simulink model "SystemModel_Working_wIntegral"  (R2014a)
settings: Solver=ode45  StartTime=0.0  StopTime=30  RelTol=1e-3
values from neighbouring files (symbols this model uses):
  a = 0.92    [SystemModelParameters_Working.m]    (also in SystemModelParameters_wIntegral_Working.m)
  b = 0.5    [SystemModelParameters_Working.m]    (also in SystemModelParameters_wIntegral_Working.m)
  initial = [10,10]    [SystemModelParameters_Working.m]    (also in SystemModelParameters_wIntegral_Working.m)
  J = 6689.281*10^-6    (= 0.006689281)    [PIDTest.m]    (also in SystemModelParameters_Working.m; SystemModelParameters_wIntegral_Working.m)
  kp = 0.0038    [PIDTest.m]    (also in SystemModelParameters_Working.m = 0.4; SystemModelParameters_wIntegral_Working.m = 0.4)
  L = (G/(1+G))    [PIDTest.m]    (also in SystemModelParameters_Working.m = 0.28484; SystemModelParameters_wIntegral_Working.m = 0.28484)
  n = 0    [PIDTest.m]    (also in SystemModelParameters_Working.m = 0.01; SystemModelParameters_wIntegral_Working.m = 0.01)
  PWMs_fixed = [1619,1638]    [SystemModelParameters_Working.m]    (also in SystemModelParameters_wIntegral_Working.m)
  Td = 2.1761/kp    (= 572.657894737)    [PIDTest.m]    (also in SystemModelParameters_Working.m = 0.578; SystemModelParameters_wIntegral_Working.m = 0.578)
  Ti = 1.1    [SystemModelParameters_wIntegral_Working.m]
  Ts = 0.02    [SystemModelParameters_wIntegral_Working.m]
undefined symbols (not defined in the file or in its folder): sigbuilder_block
libraries: aerolibconvert2 x2
settings Model: Creator=lorem  LastModifiedBy=lorem

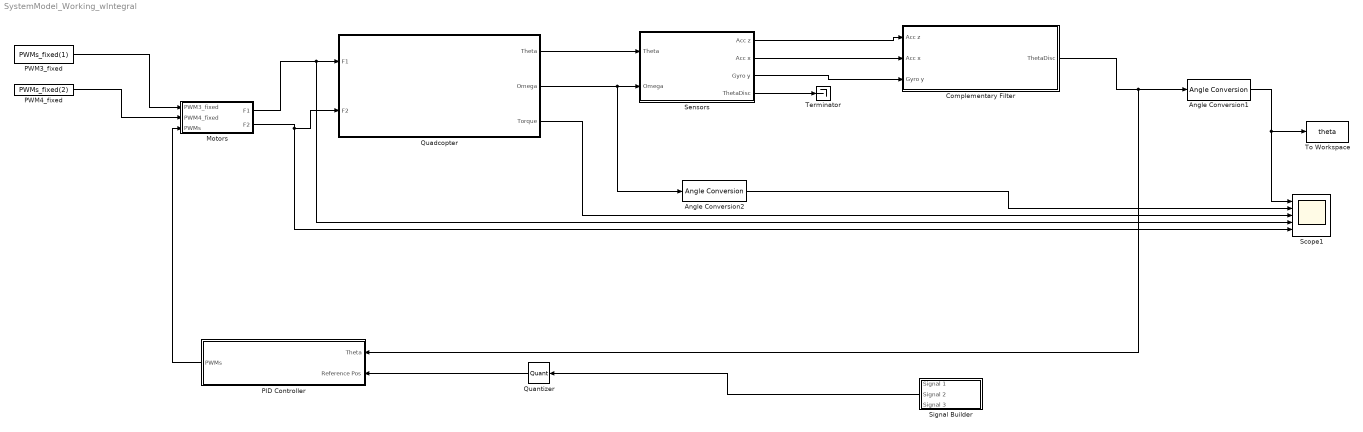
== system SystemModel_Working_wIntegral ==
  Angle Conversion1 : aerolibconvert2/Angle Conversion  IU=rad  OU=deg
  Angle Conversion2 : aerolibconvert2/Angle Conversion  IU=rad  OU=deg
  Complementary Filter : Subsystem
  Motors : Subsystem
  PID Controller : Subsystem
  PWM3_fixed : Constant  Value=PWMs_fixed(1)  SampleTime=0.02
  PWM4_fixed : Constant  Value=PWMs_fixed(2)  SampleTime=0.02
  Quadcopter : Subsystem
  Quantizer : Quantizer  QuantizationInterval=0.01  SampleTime=0.02
  Scope1 : Scope  NumInputPorts=5
      settings: TimeRange=30  YMin=-5~-5~-5~-5~-5  YMax=5~5~5~5~5
  Sensors : Subsystem
  Signal Builder : Subsystem  Tag=STV Subsys  LoadFcn=sigbuilder_block('load');  StartFcn=sigbuilder_block('start');  StopFcn=sigbuilder_block('stop');  ClipboardFcn=sigbuilder_block('clipboard');  mask(Sigbuilder block){}
      mask help: Simulink:masks:SigbuilderBlock_MD
      mask init:
      | if ~strcmp(get_param(bdroot(gcbh),'SimulationStatus'),'stopped') tuvar = sigbuilder_block('maskInit'); end
      settings: CopyFcn=sigbuilder_block('copy');  DeleteFcn=sigbuilder_block('delete');  ModelCloseFcn=sigbuilder_block('modelClose');  PreSaveFcn=sigbuilder_block('preSave');  PauseFcn=sigbuilder_block('pause');  ContinueFcn=sigbuilder_block('continue');  NameChangeFcn=sigbuilder_block('namechange');  OpenFcn=sigbuilder_block('open',[6.75 6.75 1138.5 568.5 ]);  CloseFcn=sigbuilder_block('close');
      mask Display: plot(0, 0, 100, 100,[2, 2, 32, 32, 2], [68, 8, 8, 68, 68],[32, 2], [38, 38], [32, 19, 2],[53, 60, 44], [32, 17, 17, 2],[16, 16, 31, 31]);txt = getActiveGroup(gcbh);text(2, 100, txt,'verticalAlignment', 'top');
  Terminator : Terminator
  To Workspace : ToWorkspace  VariableName=theta  SaveFormat=Timeseries  SampleTime=-1
  wires:
  PWM4_fixed/1 -> Motors/2(PWM4_fixed)
  Motors/2(F2) -> Scope1/5, Quadcopter/2(F2)
  Motors/1(F1) -> Scope1/4, Quadcopter/1(F1)
  Sensors/3(Gyro y) -> Complementary Filter/3(Gyro y)
  Sensors/2(Acc x) -> Complementary Filter/2("Acc x ")
  Sensors/1(Acc z) -> Complementary Filter/1(Acc z)
  PWM3_fixed/1 -> Motors/1(PWM3_fixed)
  PID Controller/1(PWMs) -> Motors/3(PWMs)
  Angle Conversion1/1 -> Scope1/1, To Workspace/1
  Quadcopter/2(Omega) -> Angle Conversion2/1, Sensors/2(Omega)
  Quadcopter/1(Theta) -> Sensors/1(Theta)
  Quadcopter/3("Torque ") -> Scope1/3
  Signal Builder/2(Signal 2) -> Quantizer/1
  Quantizer/1 -> PID Controller/2(Reference Pos)
  Sensors/4(ThetaDisc) -> Terminator/1
  Complementary Filter/1(ThetaDisc) -> PID Controller/1("Theta "), Angle Conversion1/1
  Angle Conversion2/1 -> Scope1/2

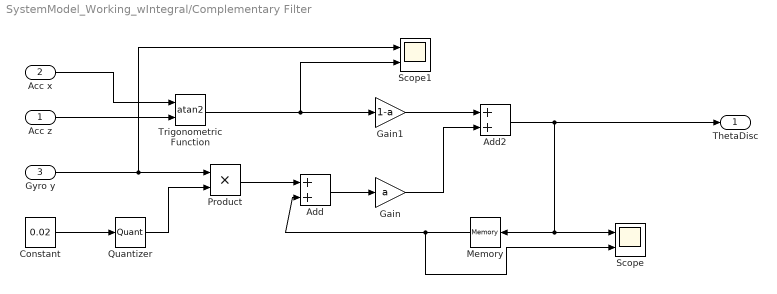
== system SystemModel_Working_wIntegral/Complementary Filter ==
  Acc z : Inport
  "Acc x " : Inport  Port=2
  Gyro y : Inport  Port=3
  Add : Sum
  Add2 : Sum
  Constant : Constant  Value=0.02
  Gain : Gain  Gain=a
  Gain1 : Gain  Gain=1-a
  Memory : Memory  X0=deg2rad(initial(2))  InheritSampleTime=on  LinearizeAsDelay=on
  Product : Product
  Quantizer : Quantizer  QuantizationInterval=0.01  SampleTime=0.02
  Scope : Scope  NumInputPorts=2
      settings: YMin=-5~-5  YMax=5~5  SaveName=ScopeData4
  Scope1 : Scope  NumInputPorts=2
      settings: YMin=-5~-5  YMax=5~5  SaveName=ScopeData5
  Trigonometric Function : Trigonometry  Operator=atan2
  ThetaDisc : Outport
  wires:
  "Acc x "/1 -> Trigonometric Function/1
  Acc z/1 -> Trigonometric Function/2
  Constant/1 -> Quantizer/1
  Gyro y/1 -> Scope1/1, Product/1
  Quantizer/1 -> Product/2
  Product/1 -> Add/1
  Add/1 -> Gain/1
  Gain1/1 -> Add2/1
  Gain/1 -> Add2/2
  Add2/1 -> ThetaDisc/1, Scope/1, Memory/1
  Memory/1 -> Scope/2, Add/2
  Trigonometric Function/1 -> Gain1/1, Scope1/2

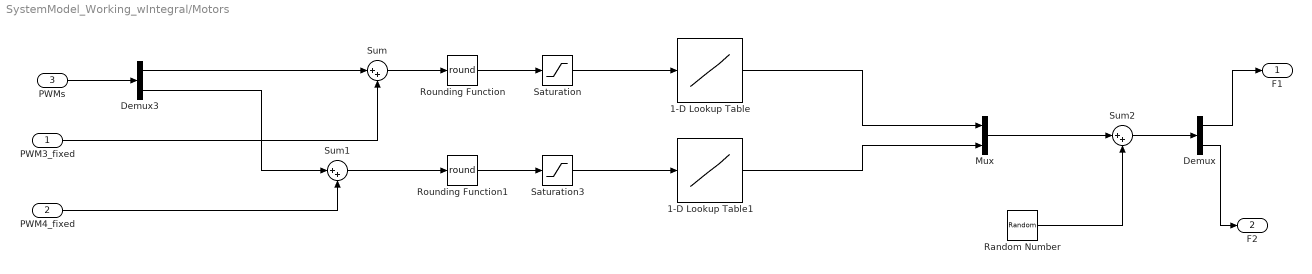
== system SystemModel_Working_wIntegral/Motors ==
  PWM3_fixed : Inport
  PWM4_fixed : Inport  Port=2
  PWMs : Inport  Port=3
  1-D Lookup Table : Lookup_n-D  NumberOfTableDimensions=1  BreakpointsForDimension1=[1447,1792]  Table=[1,5]  InternalRulePriority=Speed  RndMeth=Simplest  InputSameDT=on
  1-D Lookup Table1 : Lookup_n-D  NumberOfTableDimensions=1  BreakpointsForDimension1=[1455,1832]  Table=[1,5]  InternalRulePriority=Speed  RndMeth=Simplest  InputSameDT=on
  Demux : Demux  Outputs=2
  Demux3 : Demux  Outputs=2
  Mux : Mux  Inputs=2
  Random Number : RandomNumber  Variance=0.036579  SampleTime=0.02
  Rounding Function : Rounding  Operator=round
  Rounding Function1 : Rounding  Operator=round
  Saturation : Saturate  UpperLimit=1792  LowerLimit=1447
  Saturation3 : Saturate  UpperLimit=1832  LowerLimit=1455
  Sum : Sum  Inputs=|++
  Sum1 : Sum  Inputs=|++
  Sum2 : Sum  Inputs=|++
  F1 : Outport
  F2 : Outport  Port=2
  wires:
  PWMs/1 -> Demux3/1
  PWM4_fixed/1 -> Sum1/2
  PWM3_fixed/1 -> Sum/2
  Demux3/1 -> Sum/1
  Demux3/2 -> Sum1/1
  Sum1/1 -> Rounding Function1/1
  Rounding Function1/1 -> Saturation3/1
  Sum/1 -> Rounding Function/1
  Rounding Function/1 -> Saturation/1
  Saturation/1 -> 1-D Lookup Table/1
  Saturation3/1 -> 1-D Lookup Table1/1
  1-D Lookup Table/1 -> Mux/1
  1-D Lookup Table1/1 -> Mux/2
  Mux/1 -> Sum2/1
  Random Number/1 -> Sum2/2
  Sum2/1 -> Demux/1
  Demux/2 -> F2/1
  Demux/1 -> F1/1

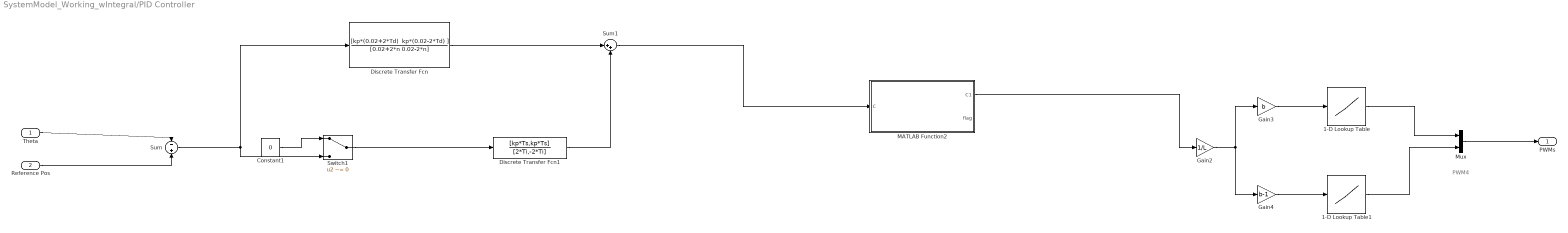
== system SystemModel_Working_wIntegral/PID Controller ==
  note: PWM4
  "Theta " : Inport
  Reference Pos : Inport  Port=2
  1-D Lookup Table : Lookup_n-D  NumberOfTableDimensions=1  BreakpointsForDimension1=[-2,2]  Table=[-138,138]  InternalRulePriority=Speed  RndMeth=Simplest  InputSameDT=on
  1-D Lookup Table1 : Lookup_n-D  NumberOfTableDimensions=1  BreakpointsForDimension1=[-2,2]  Table=[-150.8,150.8]  InternalRulePriority=Speed  RndMeth=Simplest  InputSameDT=on
  Constant1 : Constant  Value=0  SampleTime=0.02
  Discrete Transfer Fcn : DiscreteTransferFcn  Numerator="[kp*(0.02+2*Td)  kp*(0.02-2*Td) ]"  Denominator=[0.02+2*n 0.02-2*n]  SampleTime=0.02
  Discrete Transfer Fcn1 : DiscreteTransferFcn  Numerator=[kp*Ts,kp*Ts]  Denominator=[2*Ti,-2*Ti]
  Gain2 : Gain  Gain=1/L
  Gain3 : Gain  Gain=b
  Gain4 : Gain  Gain=b-1
  MATLAB Function2 : MATLAB Function  TreatAsAtomicUnit=on
  Mux : Mux  Inputs=2
  Sum : Sum  Inputs=-+
  Sum1 : Sum  Inputs=|++
  Switch1 : Switch  Criteria=u2 ~= 0
  PWMs : Outport
  wires:
  Mux/1 -> PWMs/1
  Gain4/1 -> 1-D Lookup Table1/1
  Gain3/1 -> 1-D Lookup Table/1
  Gain2/1 -> Gain3/1, Gain4/1
  1-D Lookup Table1/1 -> Mux/2
  "Theta "/1 -> Sum/1
  1-D Lookup Table/1 -> Mux/1
  Reference Pos/1 -> Sum/2
  Discrete Transfer Fcn/1 -> Sum1/1
  Sum/1 -> Switch1/3, Discrete Transfer Fcn/1
  Discrete Transfer Fcn1/1 -> Sum1/2
  Switch1/1 -> Discrete Transfer Fcn1/1
  Constant1/1 -> Switch1/1
  MATLAB Function2/1(C1) -> Gain2/1
  Sum1/1 -> MATLAB Function2/1(C)

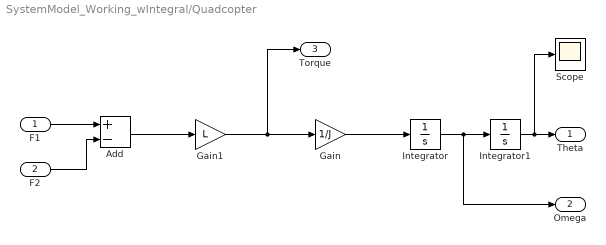
== system SystemModel_Working_wIntegral/Quadcopter ==
  F1 : Inport
  F2 : Inport  Port=2
  Add : Sum  Inputs=+-
  Gain : Gain  Gain=1/J
  Gain1 : Gain  Gain=L
  Integrator : Integrator  InitialCondition=deg2rad(initial(1))
  Integrator1 : Integrator  InitialCondition=deg2rad(initial(2))
  Scope : Scope
      settings: SaveName=ScopeData6
  Theta : Outport
  Omega : Outport  Port=2
  "Torque " : Outport  Port=3
  wires:
  Gain/1 -> Integrator/1
  Integrator/1 -> Omega/1, Integrator1/1
  F2/1 -> Add/2
  F1/1 -> Add/1
  Add/1 -> Gain1/1
  Gain1/1 -> "Torque "/1, Gain/1
  Integrator1/1 -> Scope/1, Theta/1

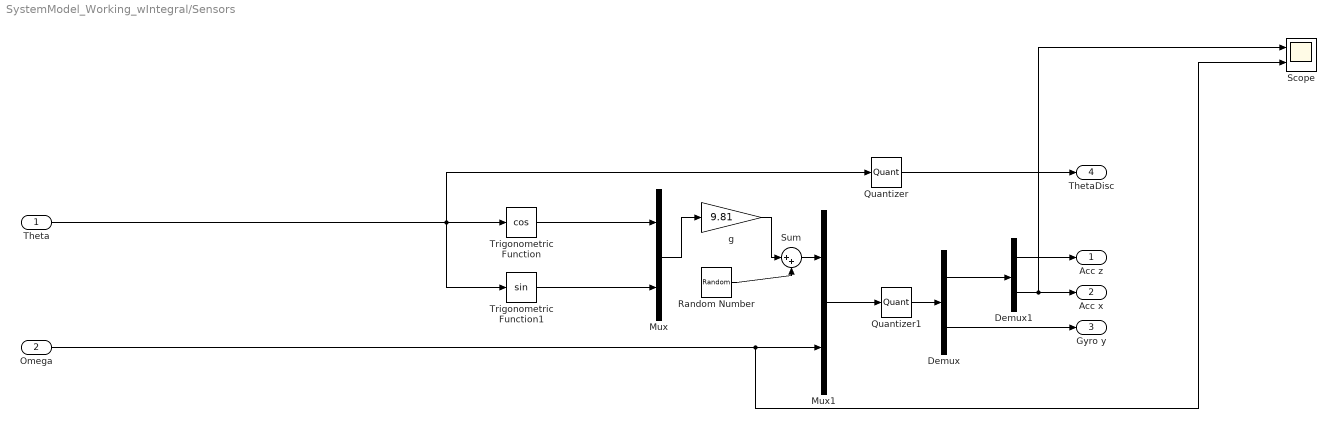
== system SystemModel_Working_wIntegral/Sensors ==
  Theta : Inport
  Omega : Inport  Port=2
  Demux : Demux  Outputs=2
  Demux1 : Demux  Outputs=2
  Mux : Mux  Inputs=2
  Mux1 : Mux  Inputs=2
  Quantizer : Quantizer  QuantizationInterval=0.01  SampleTime=0.02
  Quantizer1 : Quantizer  QuantizationInterval=0.01  SampleTime=0.02
  Random Number : RandomNumber  Variance=0.0127  SampleTime=0
  Scope : Scope  NumInputPorts=2
      settings: YMin=-5~-5  YMax=5~5  SaveName=ScopeData3
  Sum : Sum  Inputs=|++
  Trigonometric Function : Trigonometry  Operator=cos
  Trigonometric Function1 : Trigonometry
  g : Gain  Gain=9.81
  Acc z : Outport
  Acc x : Outport  Port=2
  Gyro y : Outport  Port=3
  ThetaDisc : Outport  Port=4
  wires:
  Trigonometric Function1/1 -> Mux/2
  Trigonometric Function/1 -> Mux/1
  Mux/1 -> g/1
  Mux1/1 -> Quantizer1/1
  Quantizer1/1 -> Demux/1
  Demux/2 -> Gyro y/1
  Demux/1 -> Demux1/1
  Demux1/1 -> Acc z/1
  Omega/1 -> Scope/2, Mux1/2
  Theta/1 -> Quantizer/1, Trigonometric Function1/1, Trigonometric Function/1
  Demux1/2 -> Scope/1, Acc x/1
  Quantizer/1 -> ThetaDisc/1
  g/1 -> Sum/1
  Random Number/1 -> Sum/2
  Sum/1 -> Mux1/1

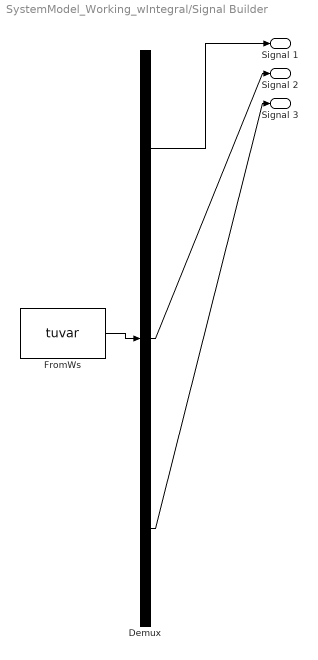
== system SystemModel_Working_wIntegral/Signal Builder ==
  Demux : Demux  Tag=STV Demux  Outputs=3
  FromWs : FromWorkspace  Tag=STV FromWs  VariableName=tuvar  SampleTime=0
      SigBuilderData=|
      | common.afterFinalStr = 'Extrapolate'
      | common.sampleTime = 0
      | dataSet.timeRange = [0 10]
      | dataSet.name = 'Group 1'
      | sbobj.Groups.Name = 'Group 1'
      | sbobj.Groups.Signals(1).Name = 'Signal 1'
      | sbobj.Groups.Signals(1).XData = [0 10]
      | sbobj.Groups.Signals(1).YData = [0 0]
      | sbobj.Groups.Signals(2).Name = 'Signal 2'
      | sbobj.Groups.Signals(2).XData = [0 5 5 10]
      | sbobj.Groups.Signals(2).YData = [0 0 1 1]
      | sbobj.Groups.Signals(3).Name = 'Signal 3'
      | sbobj.Groups.Signals(3).XData = [0 5 5 7 7 10]
      | sbobj.Groups.Signals(3).YData = [0 0 1 1 0 0]
  Signal 1 : Outport  Tag=STV Outport
  Signal 2 : Outport  Tag=STV Outport  Port=2
  Signal 3 : Outport  Tag=STV Outport  Port=3
  wires:
  Demux/1 -> Signal 1/1
  FromWs/1 -> Demux/1
  Demux/2 -> Signal 2/1
  Demux/3 -> Signal 3/1

== matlab function SystemModel_Working_wIntegral/PID Controller/MATLAB Function2 ==
  data: C1 output; flag output; C input
function [C1,flag]  = fcn(C)
flag=0;
if C>4*0.28484 || C<-4*0.28484
    flag=1;
    
end
C1=C;
end
